simulink model "Problem2"  (R2018a)
settings: Solver=VariableStepAuto  StartTime=0.0  StopTime=10.0  RelTol=1e-3
values from neighbouring files (symbols this model uses):
  b = 2    [Assignment5.m]    (also in Assignment5Problem2.m = 0; Assignment5Problem2CriticallyDamped.m = 4; Assignment5Problem2Overdamped.m = 8; Assignment5Problem2Undamped.m = 0)
  J = 2    [Assignment5.m]    (also in Assignment5Problem2.m; Assignment5Problem2CriticallyDamped.m; Assignment5Problem2Overdamped.m; Assignment5Problem2Undamped.m)
  k = 2    [Assignment5.m]    (also in Assignment5Problem2.m; Assignment5Problem2CriticallyDamped.m; Assignment5Problem2Overdamped.m; Assignment5Problem2Undamped.m)
settings Model: Creator=User  LastModifiedBy=User

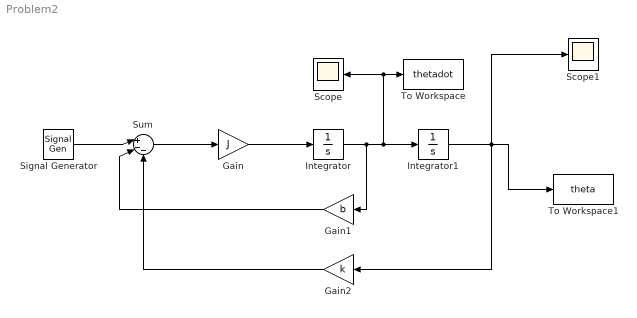
== system Problem2 ==
  Gain : Gain  Gain=J
  Gain1 : Gain  Gain=b
  Gain2 : Gain  Gain=k
  Integrator : Integrator
  Integrator1 : Integrator
  Scope : Scope
  Scope1 : Scope
  Signal Generator : SignalGenerator  Units=rad/sec
  Sum : Sum  Inputs=|+--
  To Workspace : ToWorkspace  VariableName=thetadot  SaveFormat=Timeseries  SampleTime=-1
  To Workspace1 : ToWorkspace  VariableName=theta  SaveFormat=Timeseries  SampleTime=-1
  wires:
  Gain/1 -> Integrator/1
  Integrator/1 -> Integrator1/1, Scope/1, To Workspace/1, Gain1/1
  Sum/1 -> Gain/1
  Signal Generator/1 -> Sum/1
  Gain1/1 -> Sum/2
  Gain2/1 -> Sum/3
  Integrator1/1 -> Gain2/1, Scope1/1, To Workspace1/1
